simulink model "mysysIM"  (R2019a)
settings: Solver=VariableStepAuto  StartTime=0.0  StopTime=simTime  RelTol=1e-3
values from neighbouring files (symbols this model uses):
  delta = 30    [main.m]
undefined symbols (not defined in the file or in its folder): a, A, b
settings Model: Creator=lzr96  LastModifiedBy=lzr96
settings DataIOCC: ReturnWorkspaceOutputs=off

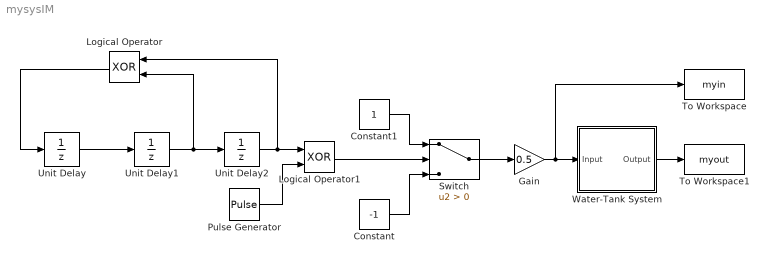
== system mysysIM ==
  Constant : Constant  Value=-1
  Constant1 : Constant
  Gain : Gain  Gain=0.5
  Logical Operator : Logic  Operator=XOR  AllPortsSameDT=off  OutDataTypeStr=boolean
  Logical Operator1 : Logic  Operator=XOR  AllPortsSameDT=off  OutDataTypeStr=boolean
  Pulse Generator : DiscretePulseGenerator  PulseType=Time based  Period=delta*2  PulseWidth=50
  Switch : Switch  Criteria=u2 > Threshold
  To Workspace : ToWorkspace  VariableName=myin  SampleTime=delta
  To Workspace1 : ToWorkspace  VariableName=myout  SampleTime=delta
  Unit Delay : UnitDelay  InitialCondition=1  SampleTime=delta  HasFrameUpgradeWarning=on
  Unit Delay1 : UnitDelay  SampleTime=delta  HasFrameUpgradeWarning=on
  Unit Delay2 : UnitDelay  InitialCondition=1  SampleTime=delta  HasFrameUpgradeWarning=on
  Water-Tank System : Subsystem
      mask Display: image('1.bmp');
  wires:
  Constant/1 -> Switch/3
  Logical Operator/1 -> Unit Delay/1
  Constant1/1 -> Switch/1
  Unit Delay/1 -> Unit Delay1/1
  Switch/1 -> Gain/1
  Unit Delay1/1 -> Logical Operator/2, Unit Delay2/1
  Gain/1 -> Water-Tank System/1(Input), To Workspace/1
  Unit Delay2/1 -> Logical Operator1/1, Logical Operator/1
  Pulse Generator/1 -> Logical Operator1/2
  Logical Operator1/1 -> Switch/2
  Water-Tank System/1(Output) -> To Workspace1/1

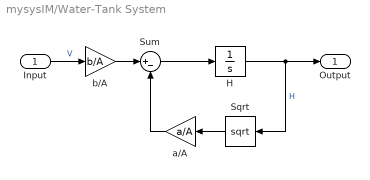
== system mysysIM/Water-Tank System ==
  Input : Inport
  H : Integrator  InitialCondition=1
  Sqrt : Sqrt  OutputSignalType=real  SaturateOnIntegerOverflow=on
  Sum : Sum  Inputs=|+-  SaturateOnIntegerOverflow=on
  a/A : Gain  Gain=a/A  SaturateOnIntegerOverflow=on  OutDataTypeStr=Inherit: Same as input  ParamDataTypeStr=Inherit: Same as input
  b/A : Gain  Gain=b/A  SaturateOnIntegerOverflow=on  OutDataTypeStr=Inherit: Same as input  ParamDataTypeStr=Inherit: Same as input
  Output : Outport
  wires:
  b/A/1 -> Sum/1
  Sum/1 -> H/1
  H/1 -> Sqrt/1, Output/1  "H"
  Sqrt/1 -> a/A/1
  a/A/1 -> Sum/2
  Input/1 -> b/A/1  "V"
